simulink model "threephaseinverter180"  (R2015b)
settings: Solver=VariableStepAuto  StartTime=0.0  StopTime=10  FixedStep=0.001  RelTol=1e-3
values from neighbouring files (symbols this model uses):
  ts = 0.001    [initial_states.m]
  Vdc = 582    [initial_states.m]
undefined symbols (not defined in the file or in its folder): j
libraries: powerlib x1
settings Model: Creator=hp  LastModifiedBy=deepika
settings DataIOCC: SaveFormat=Array  SignalLoggingSaveFormat=ModelDataLogs
settings OptimizationCC: ExpressionDepthLimit=2147483647
settings DebuggingCC: ReadBeforeWriteMsg=EnableAllAsError  WriteAfterWriteMsg=EnableAllAsError  WriteAfterReadMsg=EnableAllAsError  UnderspecifiedInitializationDetection=Classic  MergeDetectMultiDrivingBlocksExec=none  MaxConsecutiveZCsMsg=none  FcnCallInpInsideContextMsg=EnableAllAsWarning  AllowSymbolicDim=on  StateNameClashWarn=warning
settings HardwareCC: ProdBitPerPointer=32  ProdLargestAtomicFloat=None  ProdIntDivRoundTo=Undefined  ProdEndianess=Unspecified  ProdWordSize=32  ProdHWDeviceType=32-bit Generic
settings GRTTargetCC: GeneratePreprocessorConditionals=Disable all  CombineOutputUpdateFcns=off  GRTInterface=on
settings ConfigComp: CovModelRefEnable=Off

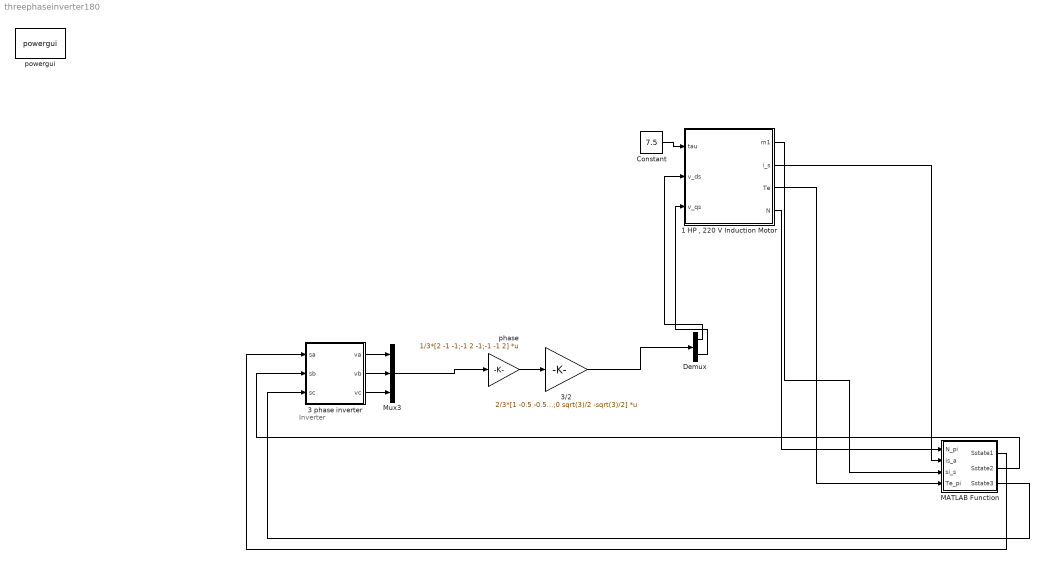
== system threephaseinverter180 ==
  note: Inverter
  "1 HP , 220 V Induction Motor" : Subsystem  mask(Induction Motor: By SRIKANTH D){Rs=10.1, Ls=(15.81+245.8954)/(2*pi*50), Rr=9.8546, Lr=(15.81+245.8954)/(2*pi*50), Lm=(245.8954)/(2*pi*50), J=0.0088, P=4}
      mask prompts: Rs "Stator Resistance  Rs [ohms] :"; Ls "Stator Inductance Ls [Hendry] :"; Rr "Rotor Resistance Rr [ohms] :"; Lr "Rotor Inductance Lr [Hendry] :"; Lm "Mutual Inductance Lm [Hendry] :"; J "Rotor Inertia J [Kg-m2] :"; P "Number of Poles p :"
      mask help: Dynamic Modelling of Induction by using Mathematic Equations
      mask Display: fprintf('Induction\nMotor')
  3 phase inverter : Subsystem
  3/2 : Gain  Gain=2/3*[1 -0.5 -0.5;0 sqrt(3)/2 -sqrt(3)/2]  Multiplication=Matrix(K*u)  SaturateOnIntegerOverflow=on  OutDataTypeStr=Inherit: Same as input  ParamDataTypeStr=Inherit: Same as input
  Constant : Constant  Value=7.5
  Demux : Demux  Outputs=2
  MATLAB Function : MATLAB Function  TreatAsAtomicUnit=on
  Mux3 : Mux  Inputs=3
  phase : Gain  Gain=1/3*[2 -1 -1;-1 2 -1;-1 -1 2]  Multiplication=Matrix(K*u)  SaturateOnIntegerOverflow=on  OutDataTypeStr=Inherit: Same as input  ParamDataTypeStr=Inherit: Same as input
  powergui : powerlib/powergui  Priority=1  SimulationMode=Discrete  SolverType=Tustin/Backward Euler (TBE)  SampleTime=0.001  frequency=60  SPID=off  DisableSnubberDevices=off  DisableRonSwitches=off  DisableVfSwitches=off  SwTol=0  DisplayEquations=off  Interpol=off  ExternalGateDelay=off  methode=off  Ts=100  FunctionMessages=off  echomessages=off  HookPort=off  EnableUseOfTLC=off  x0status=blocks  frequencyindice=0  Pbase=100e6  ErrMax=1e-4  Iterations=50  UnitsV=kV  UnitsW=MW  buscounter=0  RestoreLinks=warning  ResistiveCurrentMeasurement=off  Frange=[0:2:500]  Ylog=off  Xlog=on  ShowGrid=off  save=off  variable=ZData  structure=0  ZoomFFT=off  StartTime=0.0  cycles=1  DisplayStyle=1  fundamental=60  FreqAxis=off  MaxFrequency=1000  frequencyindicesteady=1  RmsSteady=1  display=off
  wires:
  Constant/1 -> "1 HP , 220 V Induction Motor"/1(tau)
  "1 HP , 220 V Induction Motor"/1(m1) -> MATLAB Function/3(si_s)
  3/2/1 -> Demux/1
  phase/1 -> 3/2/1
  Mux3/1 -> phase/1
  Demux/1 -> "1 HP , 220 V Induction Motor"/2(v_ds)
  Demux/2 -> "1 HP , 220 V Induction Motor"/3(v_qs)
  MATLAB Function/2(Sstate2) -> 3 phase inverter/2(sb)
  MATLAB Function/1(Sstate1) -> 3 phase inverter/1(sa)
  MATLAB Function/3(Sstate3) -> 3 phase inverter/3(sc)
  3 phase inverter/1(va) -> Mux3/1
  3 phase inverter/2(vb) -> Mux3/2
  3 phase inverter/3(vc) -> Mux3/3
  "1 HP , 220 V Induction Motor"/2(i_s) -> MATLAB Function/2(is_a)
  "1 HP , 220 V Induction Motor"/3(Te) -> MATLAB Function/4(Te_pi)
  "1 HP , 220 V Induction Motor"/4(N) -> MATLAB Function/1(N_pi)

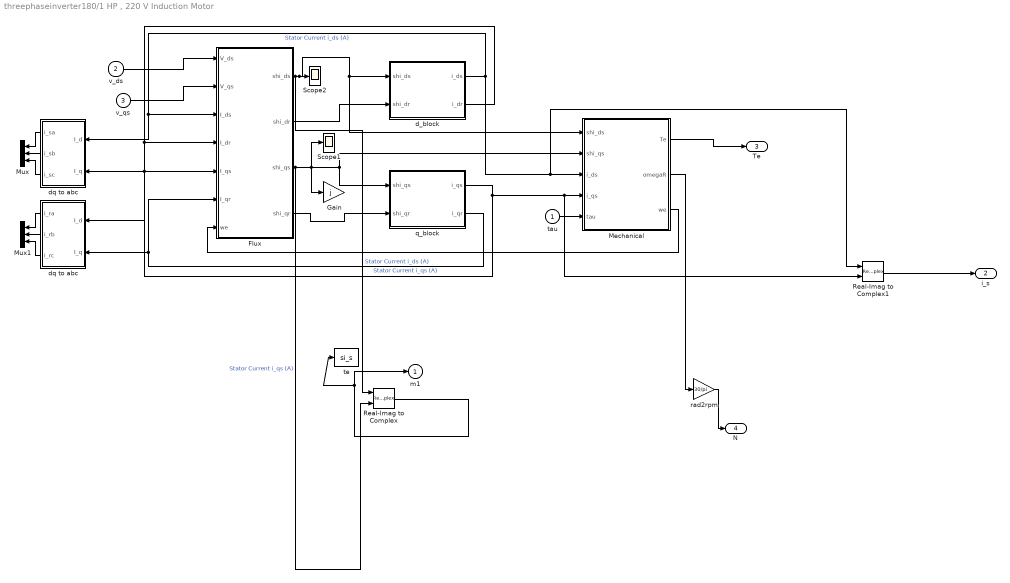
== system threephaseinverter180/1 HP , 220 V Induction Motor ==
  tau : Inport
  v_ds : Inport  Port=2
  v_qs : Inport  Port=3
  Flux : Subsystem
  Gain : Gain  Gain=j
  Mechanical : Subsystem
  Mux : Mux  Inputs=3
  Mux1 : Mux  Inputs=3
  Real-Imag to Complex : RealImagToComplex
  Real-Imag to Complex1 : RealImagToComplex
  Scope1 : Scope
  Scope2 : Scope
  d_block : Subsystem
  dq to abc : Subsystem
  "dq to abc " : Subsystem
  q_block : Subsystem
  rad2rpm : Gain  Gain=30/pi
  te : ToWorkspace  VariableName=si_s  SampleTime=ts
  m1 : Outport
  i_s : Outport  Port=2
  Te : Outport  Port=3
  N : Outport  Port=4
  wires:
  Mechanical/2(omegaR) -> rad2rpm/1
  Mechanical/3(we) -> Flux/7(we)
  Flux/4("shi_qr ") -> q_block/2(shi_qr)
  d_block/2(i_dr) -> Flux/4(I_dr), "dq to abc "/1(I_d)
  q_block/2(i_qr) -> "dq to abc "/2(I_q), Flux/6(I_qr)
  Mechanical/1(Te) -> Te/1
  tau/1 -> Mechanical/5(tau)
  Flux/2("shi_dr ") -> d_block/2(shi_dr)
  dq to abc/1(i_sa) -> Mux/1
  "dq to abc "/1(i_ra) -> Mux1/1
  dq to abc/2(i_sb) -> Mux/2
  dq to abc/3(i_sc) -> Mux/3
  "dq to abc "/3(i_rc) -> Mux1/3
  "dq to abc "/2(i_rb) -> Mux1/2
  rad2rpm/1 -> N/1
  v_qs/1 -> Flux/2(V_qs)
  v_ds/1 -> Flux/1(V_ds)
  Flux/3(shi_qs) -> Real-Imag to Complex/2, Scope1/1, Gain/1, q_block/1(shi_qs), Mechanical/2(shi_qs)  "Stator Current i_qs (A)"
  Flux/1(shi_ds) -> Real-Imag to Complex/1, d_block/1(shi_ds), Mechanical/1(shi_ds), Scope2/1  "Stator Current i_ds (A)"
  Real-Imag to Complex/1 -> m1/1, te/1
  q_block/1(i_qs) -> Real-Imag to Complex1/2, Mechanical/4(i_qs), dq to abc/2(I_q), Flux/5(I_qs)  "Stator Current i_qs (A)"
  d_block/1(i_ds) -> Real-Imag to Complex1/1, Mechanical/3(i_ds), dq to abc/1(I_d), Flux/3(I_ds)  "Stator Current i_ds (A)"
  Real-Imag to Complex1/1 -> i_s/1

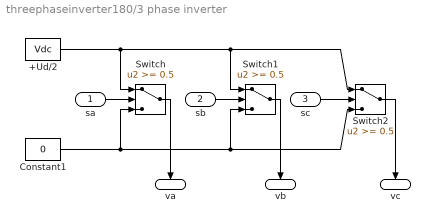
== system threephaseinverter180/3 phase inverter ==
  sa : Inport
  sb : Inport  Port=2
  sc : Inport  Port=3
  +Ud/2 : Constant  Value=Vdc
  Constant1 : Constant  Value=0
  Switch : Switch  Threshold=0.5  SaturateOnIntegerOverflow=on  InputSameDT=on
  Switch1 : Switch  Threshold=0.5  SaturateOnIntegerOverflow=on  InputSameDT=on
  Switch2 : Switch  Threshold=0.5  SaturateOnIntegerOverflow=on  InputSameDT=on
  va : Outport  InitialOutput=0
  vb : Outport  Port=2  InitialOutput=0
  vc : Outport  Port=3  InitialOutput=0
  wires:
  Switch1/1 -> vb/1
  Switch2/1 -> vc/1
  sc/1 -> Switch2/2
  sb/1 -> Switch1/2
  Switch/1 -> va/1
  sa/1 -> Switch/2
  Constant1/1 -> Switch2/3, Switch1/3, Switch/3
  +Ud/2/1 -> Switch2/1, Switch1/1, Switch/1

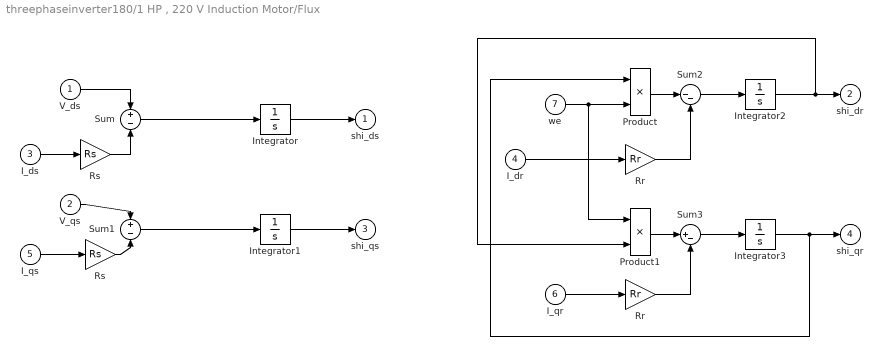
== system threephaseinverter180/1 HP , 220 V Induction Motor/Flux ==
  V_ds : Inport
  V_qs : Inport  Port=2
  I_ds : Inport  Port=3
  I_dr : Inport  Port=4
  I_qs : Inport  Port=5
  I_qr : Inport  Port=6
  we : Inport  Port=7
  Integrator{,1..3} (4 alike) : Integrator
  Product : Product
  Product1 : Product
  Rr : Gain  Gain=Rr
  "Rr " : Gain  Gain=Rr
  Rs : Gain  Gain=Rs
  "Rs " : Gain  Gain=Rs
  Sum : Sum  Inputs=+|-
  Sum1 : Sum  Inputs=+|-
  Sum2 : Sum  Inputs=|--
  Sum3 : Sum  Inputs=|+-
  shi_ds : Outport
  "shi_dr " : Outport  Port=2
  shi_qs : Outport  Port=3
  "shi_qr " : Outport  Port=4
  wires:
  Sum3/1 -> Integrator3/1
  "Rr "/1 -> Sum3/2
  Product1/1 -> Sum3/1
  I_qr/1 -> "Rr "/1
  Integrator2/1 -> "shi_dr "/1, Product1/2
  Sum2/1 -> Integrator2/1
  Product/1 -> Sum2/1
  Rr/1 -> Sum2/2
  I_dr/1 -> Rr/1
  Integrator3/1 -> "shi_qr "/1, Product/1
  we/1 -> Product1/1, Product/2
  "Rs "/1 -> Sum1/2
  Rs/1 -> Sum/2
  Integrator1/1 -> shi_qs/1
  Integrator/1 -> shi_ds/1
  Sum1/1 -> Integrator1/1
  V_qs/1 -> Sum1/1
  I_qs/1 -> "Rs "/1
  Sum/1 -> Integrator/1
  V_ds/1 -> Sum/1
  I_ds/1 -> Rs/1

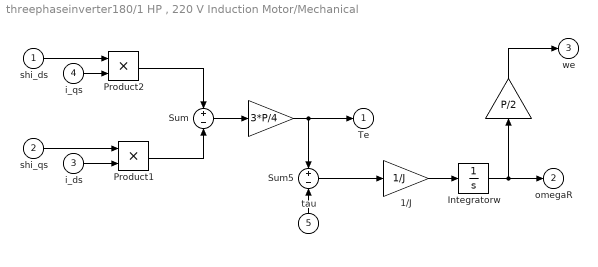
== system threephaseinverter180/1 HP , 220 V Induction Motor/Mechanical ==
  shi_ds : Inport
  shi_qs : Inport  Port=2
  i_ds : Inport  Port=3
  i_qs : Inport  Port=4
  tau : Inport  Port=5
  " " : Gain  Gain=P/2  SaturateOnIntegerOverflow=on  OutDataTypeStr=Inherit: Same as input  ParamDataTypeStr=Inherit: Same as input
  "  " : Gain  Gain=3*P/4  SaturateOnIntegerOverflow=on  OutDataTypeStr=Inherit: Same as input  ParamDataTypeStr=Inherit: Same as input
  1/J : Gain  Gain=1/J  SaturateOnIntegerOverflow=on  OutDataTypeStr=Inherit: Same as input  ParamDataTypeStr=Inherit: Same as input
  Integratorw : Integrator
  Product1 : Product
  Product2 : Product
  Sum : Sum  Inputs=+|-
  Sum5 : Sum  Inputs=+-  SaturateOnIntegerOverflow=on  InputSameDT=on  OutDataTypeStr=Inherit: Same as first input
  Te : Outport
  omegaR : Outport  Port=2
  we : Outport  Port=3
  wires:
  " "/1 -> we/1
  Integratorw/1 -> omegaR/1, " "/1
  1/J/1 -> Integratorw/1
  Sum5/1 -> 1/J/1
  tau/1 -> Sum5/2
  "  "/1 -> Sum5/1, Te/1
  Sum/1 -> "  "/1
  Product2/1 -> Sum/1
  Product1/1 -> Sum/2
  i_ds/1 -> Product1/2
  shi_qs/1 -> Product1/1
  i_qs/1 -> Product2/2
  shi_ds/1 -> Product2/1

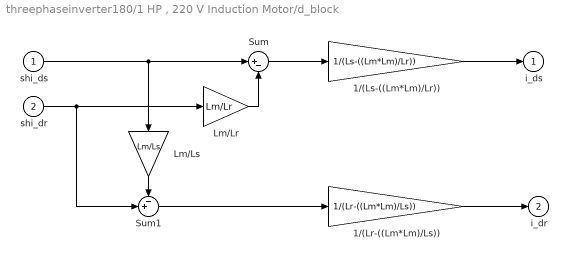
== system threephaseinverter180/1 HP , 220 V Induction Motor/d_block ==
  shi_ds : Inport
  shi_dr : Inport  Port=2
  1/(Lr-((Lm*Lm)/Ls)) : Gain  Gain=1/(Lr-((Lm*Lm)/Ls))  SaturateOnIntegerOverflow=on  OutDataTypeStr=Inherit: Same as input  ParamDataTypeStr=Inherit: Same as input
  1/(Ls-((Lm*Lm)/Lr)) : Gain  Gain=1/(Ls-((Lm*Lm)/Lr))  SaturateOnIntegerOverflow=on  OutDataTypeStr=Inherit: Same as input  ParamDataTypeStr=Inherit: Same as input
  Lm/Lr : Gain  Gain=Lm/Lr
  Lm/Ls : Gain  Gain=Lm/Ls
  Sum : Sum  Inputs=|+-
  Sum1 : Sum  Inputs=-+|
  i_ds : Outport
  i_dr : Outport  Port=2
  wires:
  Sum1/1 -> 1/(Lr-((Lm*Lm)/Ls))/1
  Lm/Ls/1 -> Sum1/1
  Sum/1 -> 1/(Ls-((Lm*Lm)/Lr))/1
  Lm/Lr/1 -> Sum/2
  shi_dr/1 -> Sum1/2, Lm/Lr/1
  shi_ds/1 -> Lm/Ls/1, Sum/1
  1/(Lr-((Lm*Lm)/Ls))/1 -> i_dr/1
  1/(Ls-((Lm*Lm)/Lr))/1 -> i_ds/1

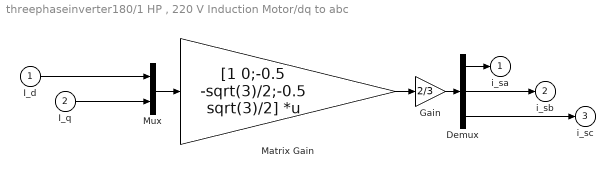
== system threephaseinverter180/1 HP , 220 V Induction Motor/dq to abc ==
  I_d : Inport
  I_q : Inport  Port=2
  Demux : Demux  Outputs=3
  Gain : Gain  Gain=2/3  SaturateOnIntegerOverflow=on  OutDataTypeStr=Inherit: Same as input  ParamDataTypeStr=Inherit: Same as input
  Matrix Gain : Gain  Gain=[1 0;-0.5 -sqrt(3)/2;-0.5 sqrt(3)/2]  Multiplication=Matrix(K*u)  SaturateOnIntegerOverflow=on  OutDataTypeStr=Inherit: Same as input  ParamDataTypeStr=Inherit: Same as input
  Mux : Mux  Inputs=2
  i_sa : Outport
  i_sb : Outport  Port=2
  i_sc : Outport  Port=3
  wires:
  Demux/1 -> i_sa/1
  Demux/3 -> i_sc/1
  I_q/1 -> Mux/2
  I_d/1 -> Mux/1
  Demux/2 -> i_sb/1
  Matrix Gain/1 -> Gain/1
  Gain/1 -> Demux/1
  Mux/1 -> Matrix Gain/1

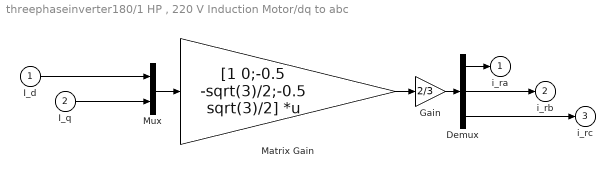
== system threephaseinverter180/1 HP , 220 V Induction Motor/dq to abc  ==
  I_d : Inport
  I_q : Inport  Port=2
  Demux : Demux  Outputs=3
  Gain : Gain  Gain=2/3  SaturateOnIntegerOverflow=on  OutDataTypeStr=Inherit: Same as input  ParamDataTypeStr=Inherit: Same as input
  Matrix Gain : Gain  Gain=[1 0;-0.5 -sqrt(3)/2;-0.5 sqrt(3)/2]  Multiplication=Matrix(K*u)  SaturateOnIntegerOverflow=on  OutDataTypeStr=Inherit: Same as input  ParamDataTypeStr=Inherit: Same as input
  Mux : Mux  Inputs=2
  i_ra : Outport
  i_rb : Outport  Port=2
  i_rc : Outport  Port=3
  wires:
  Mux/1 -> Matrix Gain/1
  Gain/1 -> Demux/1
  Matrix Gain/1 -> Gain/1
  Demux/2 -> i_rb/1
  I_d/1 -> Mux/1
  I_q/1 -> Mux/2
  Demux/3 -> i_rc/1
  Demux/1 -> i_ra/1

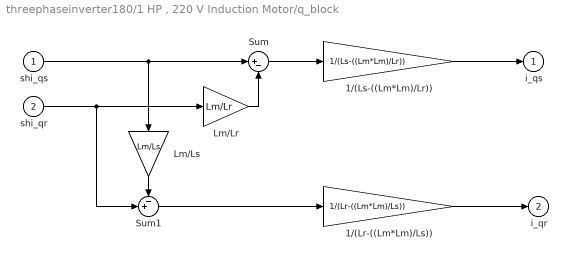
== system threephaseinverter180/1 HP , 220 V Induction Motor/q_block ==
  shi_qs : Inport
  shi_qr : Inport  Port=2
  1/(Lr-((Lm*Lm)/Ls)) : Gain  Gain=1/(Lr-((Lm*Lm)/Ls))  SaturateOnIntegerOverflow=on  OutDataTypeStr=Inherit: Same as input  ParamDataTypeStr=Inherit: Same as input
  1/(Ls-((Lm*Lm)/Lr)) : Gain  Gain=1/(Ls-((Lm*Lm)/Lr))  SaturateOnIntegerOverflow=on  OutDataTypeStr=Inherit: Same as input  ParamDataTypeStr=Inherit: Same as input
  Lm/Lr : Gain  Gain=Lm/Lr
  Lm/Ls : Gain  Gain=Lm/Ls
  Sum : Sum  Inputs=|+-
  Sum1 : Sum  Inputs=-+|
  i_qs : Outport
  i_qr : Outport  Port=2
  wires:
  Sum1/1 -> 1/(Lr-((Lm*Lm)/Ls))/1
  Lm/Ls/1 -> Sum1/1
  Sum/1 -> 1/(Ls-((Lm*Lm)/Lr))/1
  Lm/Lr/1 -> Sum/2
  shi_qr/1 -> Lm/Lr/1, Sum1/2
  shi_qs/1 -> Lm/Ls/1, Sum/1
  1/(Lr-((Lm*Lm)/Ls))/1 -> i_qr/1
  1/(Ls-((Lm*Lm)/Lr))/1 -> i_qs/1

== matlab function threephaseinverter180/MATLAB Function ==
  data: N_pi input; is_a input; Sstate1 output; si_s input; Te_pi input; Sstate2 output; Sstate3 output
function [Sstate1,    Sstate2,   Sstate3]     = fcn(N_pi, is_a, si_s, Te_pi)
%#codegen

S=[0 0 0;0 0 1; 0 1 0;0 1 1;1 0 0;1 0 1;1 1 0;1 1 1];
 
k=1;
gj=0;
Vs=[0+0j 0+0j 0+0j 0+0j 0+0j 0+0j 0+0j 0+0j];
is_a1_k1 = [0+0j 0+0j 0+0j 0+0j 0+0j 0+0j 0+0j 0+0j];
si_s1_k1 = [0+0j 0+0j 0+0j 0+0j 0+0j 0+0j 0+0j 0+0j];
Te_pi1_k1 =[0+0j 0+0j 0+0j 0+0j 0+0j 0+0j 0+0j 0+0j];
S_state=[0 0 0];

is_a1 = is_a
N_pi1 = N_pi
si_s1 = si_s

Te_pi1=Te_pi;
Vdc=582;
Rs=2.68;
Rr=2.13;
Lm=0.275;
Ls=0.2834;
Lr=0.2834;
P=1;
N_pi_nom=2772;
T_ref=7.5;
J=0.005;
ts=0.001;

lamda_1=1;
a=-inf;

sigma=1-(Lm^2)/Ls*Lr;


for i = 1:8
    
    if S(i,1)==0
    Van=(-0.5)*Vdc;
    else
        Van=(0.5)*Vdc;
    end
    if S(i,2)==0
    Vbn=(-0.5)*Vdc;
    else
        Vbn=(0.5)*Vdc;
    end
    if S(i,3)==0
    Vcn=(-0.5)*Vdc;
    else
        Vcn=(0.5)*Vdc;
    end
    
 
    Vs(i)= Van + j*(-Vbn/sqrt(3) +Vcn/sqrt(3));
    
    is_a1_k1(i)=((ts*Rr)/(sigma*Ls*Lr)-(1*j)*(ts*N_pi1)/(sigma*Ls))*si_s1+...
            (1-(ts*Rs)/(sigma*Ls)-(ts*Rs)/(sigma*Lr)+(1*j)*ts*N_pi1)*is_a1+...
            (ts/(sigma*Ls))*Vs(i);
        
    si_s1_k1(i)= si_s1+ts*Vs(i)-ts*Rs*is_a1;
    
    Te_pi1_k1(i)= 3/2*P*imag(si_s1_k1(i)*is_a1_k1(i));
    
    gj=(T_ref-Te_pi1_k1(i));
    
        if i == 1
            a = gj;
        end
        if i==1
            v=Vs(i);
        end
        if i==1
            S_state=S(1,:);
        
        end
        
        if gj<a
           
            a=gj;
            v=Vs(i);
            S_state=S(i,:);
            
           
        end
    i=i+1;
end

Sstate1=S_state(1)
Sstate2=S_state(2)
Sstate3=S_state(3)
%{
if S_state(1)==1
    amp1=5;
    amp2=0;
else
    amp1=0;
    amp2=5;
end    
if S_state(2)==1
    amp3=5;
    amp4=0;
else
    amp3=0;
    amp4=5;
end    
if S_state(3)==1
    amp5=5;
    amp6=0;
else
    amp5=0;
    amp6=5;
end    
    %}
